simulink model "v2F"  (R2014a)
settings: Solver=FixedStepDiscrete  StartTime=0.0  StopTime=10.0  FixedStep=0.1  RelTol=1e-3
settings Model: Creator=yoshi12  LastModifiedBy=yoshi12

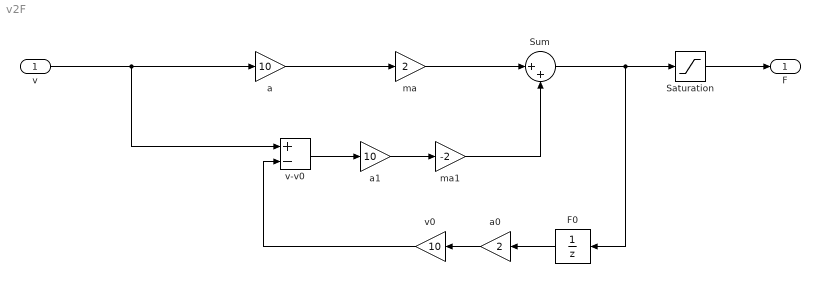
== system v2F ==
  v : Inport
  F0 : UnitDelay  SampleTime=-1
  Saturation : Saturate  UpperLimit=40  LowerLimit=-40
  Sum : Sum  Inputs=|++
  a : Gain  Gain=10
  a0 : Gain  Gain=2
  a1 : Gain  Gain=10
  ma : Gain  Gain=2
  ma1 : Gain  Gain=-2
  v-v0 : Sum  Inputs=+-
  v0 : Gain  Gain=10
  F : Outport
  wires:
  v/1 -> a/1, v-v0/1
  F0/1 -> a0/1
  ma/1 -> Sum/1
  Sum/1 -> Saturation/1, F0/1
  a/1 -> ma/1
  a0/1 -> v0/1
  v0/1 -> v-v0/2
  v-v0/1 -> a1/1
  a1/1 -> ma1/1
  ma1/1 -> Sum/2
  Saturation/1 -> F/1
